simulink model "PID_base_simulink_formigas"  (R2021b)
settings: Solver=ode23tb  StartTime=0.0  StopTime=10  RelTol=1e-3
values from neighbouring files (symbols this model uses):
  A1 = 1.2566e-3    (= 0.0012566)    [PID_Otim_formigas.m]
  A2 = 8.765e-4    (= 0.0008765)    [PID_Otim_formigas.m]
  be = 9000e5    (= 900000000)    [PID_Otim_formigas.m]
  f = 1500    [PID_Otim_formigas.m]
  g = 9.8    [PID_Otim_formigas.m]
  kc1 = 3.644e-12    [PID_Otim_formigas.m]
  kc2 = 4.376e-12    [PID_Otim_formigas.m]
  kd = k    (= 0.6684)    [PID_Otim_formigas.m]
  ki = k*z1*z2    (= 21.5599443213)    [PID_Otim_formigas.m]
  kp = k*(z1+z2)    (= 7.7681448)    [PID_Otim_formigas.m]
  kq1 = 4.76e-4    (= 0.000476)    [PID_Otim_formigas.m]
  kq2 = 4.76e-4    (= 0.000476)    [PID_Otim_formigas.m]
  M = 84    [PID_Otim_formigas.m]
  V1 = VL1+(A1*xe0)    (= 0.0001330412)    [PID_Otim_formigas.m]
  V2 = VL2+A2*(L-xe0)    (= 0.000153427)    [PID_Otim_formigas.m]
libraries: slpidlib x4, simulink x1
settings Model: Creator=cof_2  LastModifiedBy=cof_2

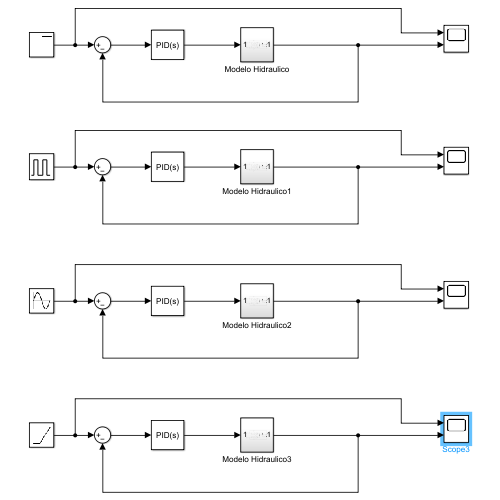
[thumbnail: Simulink's stored preview of the top-level diagram]
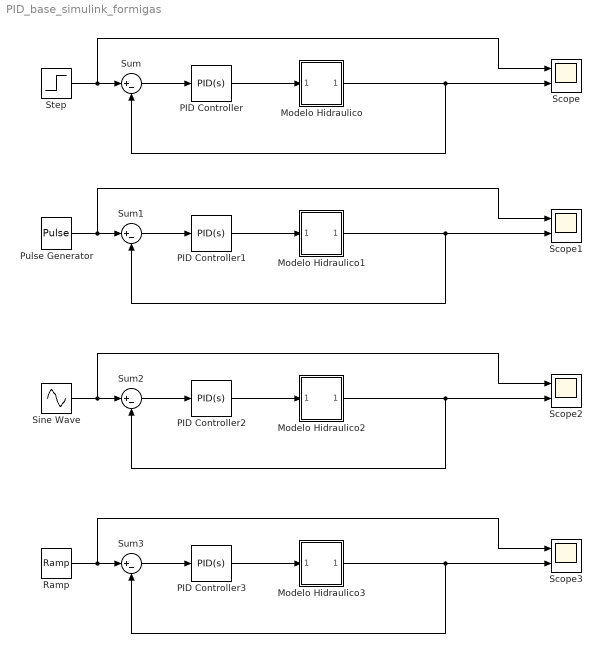
== system PID_base_simulink_formigas ==
  Modelo Hidraulico : Subsystem
  Modelo Hidraulico1 : Subsystem
  Modelo Hidraulico2 : Subsystem
  Modelo Hidraulico3 : Subsystem
  PID Controller{,1..3} (4 alike) : slpidlib/PID Controller  Controller=PID  Form=Parallel  TimeDomain=Continuous-time  UseExternalTs=off  SampleTime=-1  IntegratorMethod=Forward Euler  FilterMethod=Forward Euler  ControllerParametersSource=internal  P=kp  I=ki  D=kd  UseFilter=on  N=100  TunerSelectOption=Transfer Function Based (PID Tuner App)  InitialConditionSource=internal  InitialConditionForIntegrator=0  InitialConditionForFilter=0  DifferentiatorICPrevScaledInput=0  ExternalReset=none  TrackingMode=off  Kt=1  LimitOutput=off  SatLimitsSource=internal  UpperSaturationLimit=inf  LowerSaturationLimit=-inf  LinearizeAsGain=on  AntiWindupMode=none  Kb=1  POutMin=[]  POutMax=[]  IOutMin=[]  IOutMax=[]  DOutMin=[]  DOutMax=[]  NOutMin=[]  NOutMax=[]  SumOutMin=[]  SumOutMax=[]  SaturationOutMin=[]  SaturationOutMax=[]  PParamMin=[]  PParamMax=[]  IParamMin=[]  IParamMax=[]  DParamMin=[]  DParamMax=[]  NParamMin=[]  NParamMax=[]  KbParamMin=[]  KbParamMax=[]  KtParamMin=[]  KtParamMax=[]  KbOutMin=[]  KbOutMax=[]  KtOutMin=[]  KtOutMax=[]  IntegratorOutMin=[]  IntegratorOutMax=[]  FilterOutMin=[]  FilterOutMax=[]  SumI1OutMin=[]  SumI1OutMax=[]  SumI2OutMin=[]  SumI2OutMax=[]  SumI3OutMin=[]  SumI3OutMax=[]  SumI4OutMin=[]  SumI4OutMax=[]  SumDOutMin=[]  SumDOutMax=[]  DifferentiatorOutMin=[]  DifferentiatorOutMax=[]  FilterDiffOutCoefMin=[]  FilterDiffOutCoefMax=[]  ReciprocalOutMin=[]  ReciprocalOutMax=[]  SumDenOutMin=[]  SumDenOutMax=[]  SumNumOutMin=[]  SumNumOutMax=[]  DivideOutMin=[]  DivideOutMax=[]  UdiffTsProdOutMin=[]  UdiffTsProdOutMax=[]  NTsProdOutMin=[]  NTsProdOutMax=[]  UintegralTsProdOutMin=[]  UintegralTsProdOutMax=[]  UngainTsProdOutMin=[]  UngainTsProdOutMax=[]  FilterDenConstantOutDataTypeStr=Inherit: Inherit via back propagation  FilterDenConstantOutMin=[]  FilterDenConstantOutMax=[]  PCopyOutDataTypeStr=Inherit: Inherit via back propagation  PCopyOutMin=[]  PCopyOutMax=[]  NCopyOutDataTypeStr=Inherit: Inherit via back propagation  NCopyOutMin=[]  NCopyOutMax=[]  IntegratorContinuousStateAttributes=''  IntegratorStateMustResolveToSignalObject=off  IntegratorRTWStateStorageClass=Auto  FilterContinuousStateAttributes=''  FilterStateMustResolveToSignalObject=off  FilterRTWStateStorageClass=Auto  ParallelPVariant=InternalParameters  IdealPVariant=Disabled  IVariant=InternalParameters  DVariant=InternalParameters  IntegratorVariant=Continuous  SatVariant=Disabled  AWVariant=Passthrough  PCopyVariant=Disabled  TRVariant=Disabled  FdbkBlocksVariant=Forward  IdealPFdbkVariant=Disabled  SatFdbkVariant=Disabled  DerivativeFilterVariant=ContFilter  NVariant=InternalParameters  NCopyVariant=Disabled  FilterICVariant=InternalICsFilter  IntegratorICVariant=InternalICs  ExternalResetVariant=Disabled  TRSumVariant=Passthrough  SumFdbkVariant=Disabled  SumVariant=Sum_PID  TsampFilterVariant=InternalTs  TsampNgainVariant=Passthrough  TsampIntegralVariant=Passthrough  ExternalSaturationOutDataTypeStr=Inherit: Same as second input
  Pulse Generator : DiscretePulseGenerator  PulseType=Time based  Period=2.5  PulseWidth=5
  Ramp : simulink/Sources/Ramp  slope=1  start=0  InitialOutput=0
  Scope{,1..3} (4 alike) : Scope  NumInputPorts=2
  Sine Wave : Sin  SampleTime=0
  Step : Step  SampleTime=0
  Sum{,1..3} (4 alike) : Sum  Inputs=|+-
  wires:
  PID Controller/1 -> Modelo Hidraulico/1(In1)
  Modelo Hidraulico/1(Out1) -> Sum/2, Scope/2
  Step/1 -> Scope/1, Sum/1
  Sum/1 -> PID Controller/1
  Pulse Generator/1 -> Scope1/1, Sum1/1
  Modelo Hidraulico1/1(Out1) -> Sum1/2, Scope1/2
  PID Controller1/1 -> Modelo Hidraulico1/1(In1)
  Sum1/1 -> PID Controller1/1
  Sine Wave/1 -> Scope2/1, Sum2/1
  Modelo Hidraulico2/1(Out1) -> Sum2/2, Scope2/2
  PID Controller2/1 -> Modelo Hidraulico2/1(In1)
  Sum2/1 -> PID Controller2/1
  Ramp/1 -> Scope3/1, Sum3/1
  Modelo Hidraulico3/1(Out1) -> Sum3/2, Scope3/2
  PID Controller3/1 -> Modelo Hidraulico3/1(In1)
  Sum3/1 -> PID Controller3/1

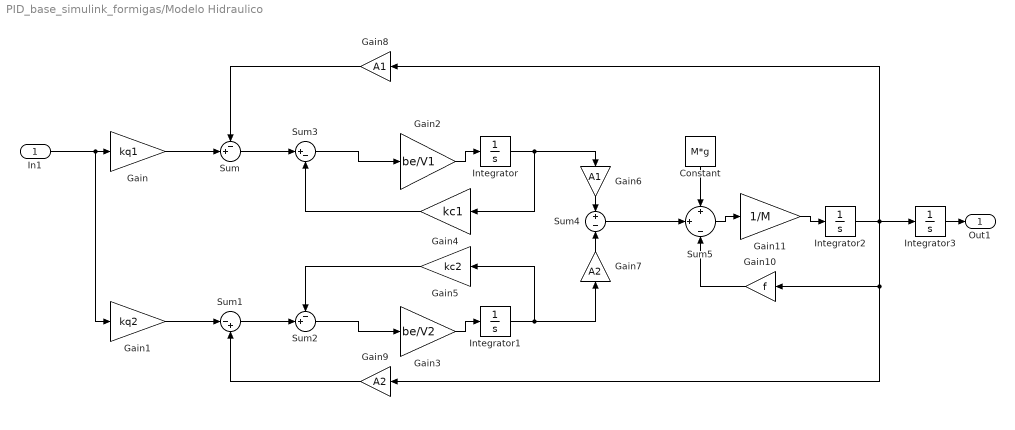
== system PID_base_simulink_formigas/Modelo Hidraulico ==
  In1 : Inport
  Constant : Constant  Value=M*g
  Gain : Gain  Gain=kq1
  Gain1 : Gain  Gain=kq2
  Gain10 : Gain  Gain=f
  Gain11 : Gain  Gain=1/M
  Gain2 : Gain  Gain=be/V1
  Gain3 : Gain  Gain=be/V2
  Gain4 : Gain  Gain=kc1
  Gain5 : Gain  Gain=kc2
  Gain6 : Gain  Gain=A1
  Gain7 : Gain  Gain=A2
  Gain8 : Gain  Gain=A1
  Gain9 : Gain  Gain=A2
  Integrator{,1..3} (4 alike) : Integrator
  Sum : Sum  Inputs=-+|
  Sum1 : Sum  Inputs=|-+
  Sum2 : Sum  Inputs=-+|
  Sum3 : Sum  Inputs=|+-
  Sum4 : Sum  Inputs=+|-
  Sum5 : Sum  Inputs=+|+|-
  Out1 : Outport
  wires:
  Sum/1 -> Sum3/1
  Constant/1 -> Sum5/1
  Sum4/1 -> Sum5/2
  Gain6/1 -> Sum4/1
  Integrator1/1 -> Gain7/1, Gain5/1
  Gain1/1 -> Sum1/1
  Integrator/1 -> Gain6/1, Gain4/1
  Sum1/1 -> Sum2/2
  Gain2/1 -> Integrator/1
  Sum5/1 -> Gain11/1
  Gain7/1 -> Sum4/2
  Gain/1 -> Sum/2
  Gain8/1 -> Sum/1
  Sum3/1 -> Gain2/1
  Integrator2/1 -> Gain8/1, Integrator3/1, Gain9/1, Gain10/1
  Gain10/1 -> Sum5/3
  Sum2/1 -> Gain3/1
  Gain5/1 -> Sum2/1
  Gain4/1 -> Sum3/2
  Gain3/1 -> Integrator1/1
  Gain9/1 -> Sum1/2
  Gain11/1 -> Integrator2/1
  In1/1 -> Gain1/1, Gain/1
  Integrator3/1 -> Out1/1

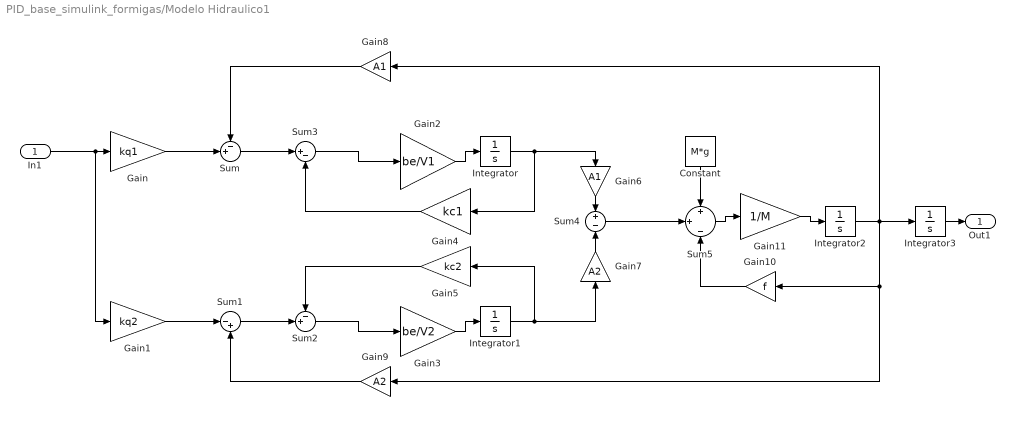
== system PID_base_simulink_formigas/Modelo Hidraulico1 ==
  In1 : Inport
  Constant : Constant  Value=M*g
  Gain : Gain  Gain=kq1
  Gain1 : Gain  Gain=kq2
  Gain10 : Gain  Gain=f
  Gain11 : Gain  Gain=1/M
  Gain2 : Gain  Gain=be/V1
  Gain3 : Gain  Gain=be/V2
  Gain4 : Gain  Gain=kc1
  Gain5 : Gain  Gain=kc2
  Gain6 : Gain  Gain=A1
  Gain7 : Gain  Gain=A2
  Gain8 : Gain  Gain=A1
  Gain9 : Gain  Gain=A2
  Integrator{,1..3} (4 alike) : Integrator
  Sum : Sum  Inputs=-+|
  Sum1 : Sum  Inputs=|-+
  Sum2 : Sum  Inputs=-+|
  Sum3 : Sum  Inputs=|+-
  Sum4 : Sum  Inputs=+|-
  Sum5 : Sum  Inputs=+|+|-
  Out1 : Outport
  wires:
  Sum/1 -> Sum3/1
  Constant/1 -> Sum5/1
  Sum4/1 -> Sum5/2
  Gain6/1 -> Sum4/1
  Integrator1/1 -> Gain7/1, Gain5/1
  Gain1/1 -> Sum1/1
  Integrator/1 -> Gain6/1, Gain4/1
  Sum1/1 -> Sum2/2
  Gain2/1 -> Integrator/1
  Sum5/1 -> Gain11/1
  Gain7/1 -> Sum4/2
  Gain/1 -> Sum/2
  Gain8/1 -> Sum/1
  Sum3/1 -> Gain2/1
  Integrator2/1 -> Gain8/1, Integrator3/1, Gain9/1, Gain10/1
  Gain10/1 -> Sum5/3
  Sum2/1 -> Gain3/1
  Gain5/1 -> Sum2/1
  Gain4/1 -> Sum3/2
  Gain3/1 -> Integrator1/1
  Gain9/1 -> Sum1/2
  Gain11/1 -> Integrator2/1
  In1/1 -> Gain1/1, Gain/1
  Integrator3/1 -> Out1/1

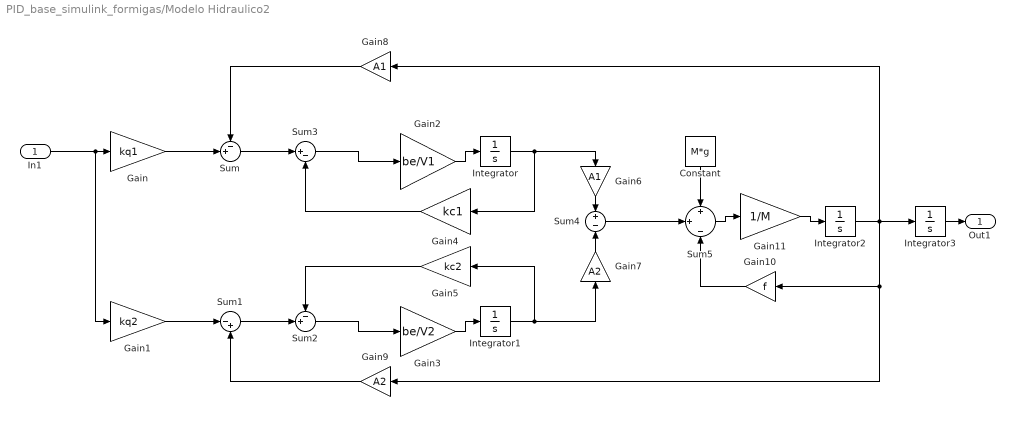
== system PID_base_simulink_formigas/Modelo Hidraulico2 ==
  In1 : Inport
  Constant : Constant  Value=M*g
  Gain : Gain  Gain=kq1
  Gain1 : Gain  Gain=kq2
  Gain10 : Gain  Gain=f
  Gain11 : Gain  Gain=1/M
  Gain2 : Gain  Gain=be/V1
  Gain3 : Gain  Gain=be/V2
  Gain4 : Gain  Gain=kc1
  Gain5 : Gain  Gain=kc2
  Gain6 : Gain  Gain=A1
  Gain7 : Gain  Gain=A2
  Gain8 : Gain  Gain=A1
  Gain9 : Gain  Gain=A2
  Integrator{,1..3} (4 alike) : Integrator
  Sum : Sum  Inputs=-+|
  Sum1 : Sum  Inputs=|-+
  Sum2 : Sum  Inputs=-+|
  Sum3 : Sum  Inputs=|+-
  Sum4 : Sum  Inputs=+|-
  Sum5 : Sum  Inputs=+|+|-
  Out1 : Outport
  wires:
  Sum/1 -> Sum3/1
  Constant/1 -> Sum5/1
  Sum4/1 -> Sum5/2
  Gain6/1 -> Sum4/1
  Integrator1/1 -> Gain7/1, Gain5/1
  Gain1/1 -> Sum1/1
  Integrator/1 -> Gain6/1, Gain4/1
  Sum1/1 -> Sum2/2
  Gain2/1 -> Integrator/1
  Sum5/1 -> Gain11/1
  Gain7/1 -> Sum4/2
  Gain/1 -> Sum/2
  Gain8/1 -> Sum/1
  Sum3/1 -> Gain2/1
  Integrator2/1 -> Gain8/1, Integrator3/1, Gain9/1, Gain10/1
  Gain10/1 -> Sum5/3
  Sum2/1 -> Gain3/1
  Gain5/1 -> Sum2/1
  Gain4/1 -> Sum3/2
  Gain3/1 -> Integrator1/1
  Gain9/1 -> Sum1/2
  Gain11/1 -> Integrator2/1
  In1/1 -> Gain1/1, Gain/1
  Integrator3/1 -> Out1/1

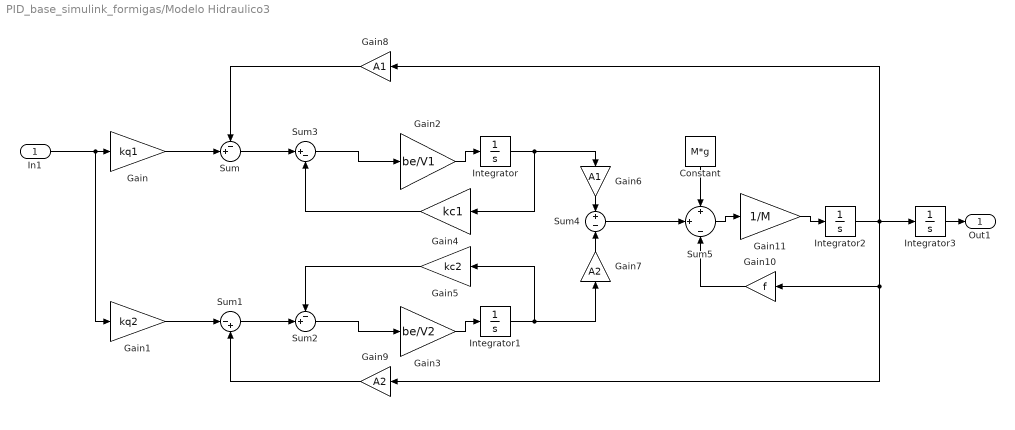
== system PID_base_simulink_formigas/Modelo Hidraulico3 ==
  In1 : Inport
  Constant : Constant  Value=M*g
  Gain : Gain  Gain=kq1
  Gain1 : Gain  Gain=kq2
  Gain10 : Gain  Gain=f
  Gain11 : Gain  Gain=1/M
  Gain2 : Gain  Gain=be/V1
  Gain3 : Gain  Gain=be/V2
  Gain4 : Gain  Gain=kc1
  Gain5 : Gain  Gain=kc2
  Gain6 : Gain  Gain=A1
  Gain7 : Gain  Gain=A2
  Gain8 : Gain  Gain=A1
  Gain9 : Gain  Gain=A2
  Integrator{,1..3} (4 alike) : Integrator
  Sum : Sum  Inputs=-+|
  Sum1 : Sum  Inputs=|-+
  Sum2 : Sum  Inputs=-+|
  Sum3 : Sum  Inputs=|+-
  Sum4 : Sum  Inputs=+|-
  Sum5 : Sum  Inputs=+|+|-
  Out1 : Outport
  wires:
  Sum/1 -> Sum3/1
  Constant/1 -> Sum5/1
  Sum4/1 -> Sum5/2
  Gain6/1 -> Sum4/1
  Integrator1/1 -> Gain7/1, Gain5/1
  Gain1/1 -> Sum1/1
  Integrator/1 -> Gain6/1, Gain4/1
  Sum1/1 -> Sum2/2
  Gain2/1 -> Integrator/1
  Sum5/1 -> Gain11/1
  Gain7/1 -> Sum4/2
  Gain/1 -> Sum/2
  Gain8/1 -> Sum/1
  Sum3/1 -> Gain2/1
  Integrator2/1 -> Gain8/1, Integrator3/1, Gain9/1, Gain10/1
  Gain10/1 -> Sum5/3
  Sum2/1 -> Gain3/1
  Gain5/1 -> Sum2/1
  Gain4/1 -> Sum3/2
  Gain3/1 -> Integrator1/1
  Gain9/1 -> Sum1/2
  Gain11/1 -> Integrator2/1
  In1/1 -> Gain1/1, Gain/1
  Integrator3/1 -> Out1/1
